simulink model "controle_discreto_pc"  (R2022a)
settings: Solver=FixedStepDiscrete  StartTime=0.0  StopTime=30  FixedStep=delta_time  RelTol=1e-3
undefined symbols (not defined in the file or in its folder): Cden, Cnum, Hden, Hnum, sym2poly
settings Model: Creator=phcs  LastModifiedBy=phcs

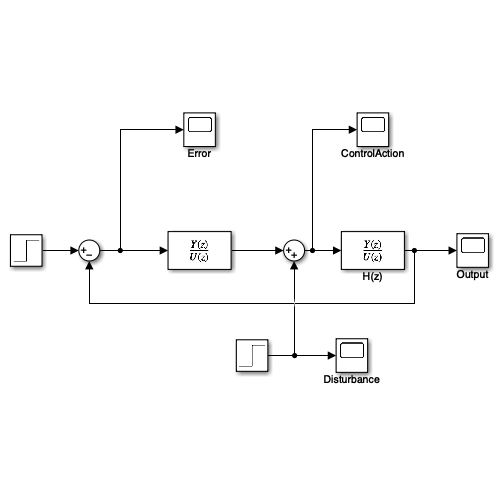
[thumbnail: Simulink's stored preview of the top-level diagram]
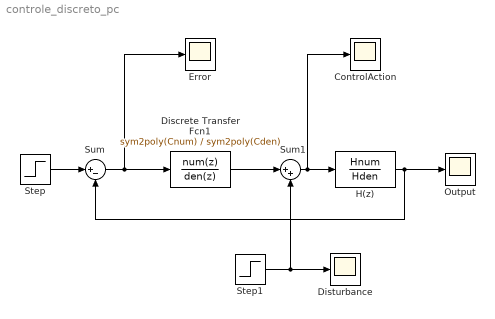
== system controle_discreto_pc ==
  ControlAction : Scope
  Discrete Transfer Fcn1 : DiscreteTransferFcn  Numerator=sym2poly(Cnum)  Denominator=sym2poly(Cden)
  Disturbance : Scope
  Error : Scope
  H(z) : DiscreteTransferFcn  Numerator=Hnum  Denominator=Hden
  Output : Scope
  Step : Step  After=3  SampleTime=0
  Step1 : Step  Time=10  SampleTime=0
  Sum : Sum  Inputs=|+-
  Sum1 : Sum  Inputs=|++
  wires:
  H(z)/1 -> Sum/2, Output/1
  Sum/1 -> Discrete Transfer Fcn1/1, Error/1
  Step/1 -> Sum/1
  Sum1/1 -> H(z)/1, ControlAction/1
  Discrete Transfer Fcn1/1 -> Sum1/1
  Step1/1 -> Disturbance/1, Sum1/2
